simulink subsystem "EncodersAJ"  (R2023b)
settings: Solver=VariableStepAuto  StartTime=0.0  StopTime=10.0  RelTol=1e-3
libraries: arduinosensorlib x2
settings Model: Creator=jaime  LastModifiedBy=jaime

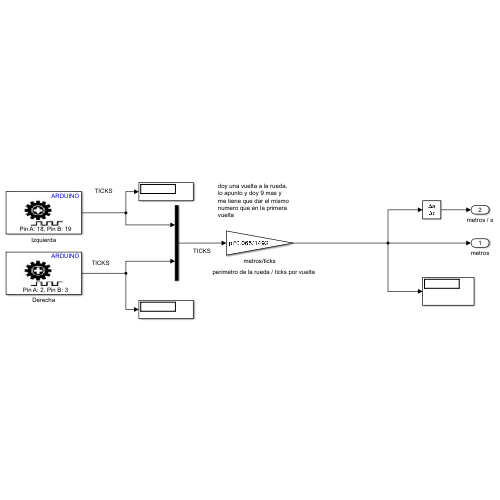
[thumbnail: Simulink's stored preview of the top-level diagram]
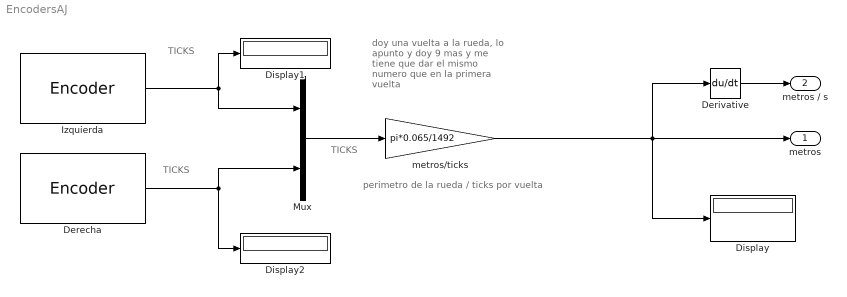
== system EncodersAJ ==
  note: TICKS
  note: TICKS
  note: TICKS
  note: perimetro de la rueda / ticks por vuelta
  note: doy una vuelta a la rueda, lo apunto y doy 9 mas y me tiene que dar el mismo numero que en la primera vuelta
  Derecha : arduinosensorlib/Encoder  InputA=2  InputB=3  Mode=No reset  SampleTime=-1
  Derivative : Derivative
  Display : Display
  Display1 : Display
  Display2 : Display
  Izquierda : arduinosensorlib/Encoder  InputA=18  InputB=19  Mode=No reset  SampleTime=-1
  Mux : Mux  Inputs=2
  metros/ticks : Gain  Gain=pi*0.065/1492  OutDataTypeStr=double
  metros : Outport
  metros / s : Outport  Port=2
  wires:
  metros/ticks/1 -> Display/1, Derivative/1, metros/1
  Derecha/1 -> Display2/1, Mux/2
  Derivative/1 -> metros / s/1
  Mux/1 -> metros/ticks/1
  Izquierda/1 -> Display1/1, Mux/1
